simulink model "test"  (R2019b)
settings: Solver=VariableStepAuto  StartTime=0.0  StopTime=10.0  RelTol=1e-3
undefined symbols (not defined in the file or in its folder): SignalState

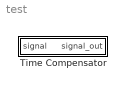
== system test ==
  Time Compensator : Subsystem  AncestorBlock=helperlibrary/Time Compensator  TreatAsAtomicUnit=on

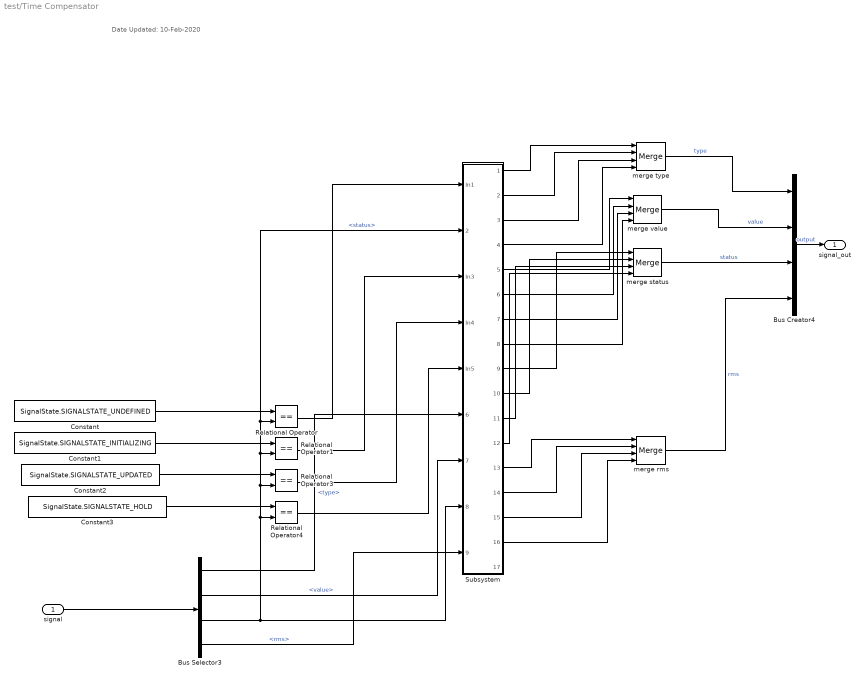
== system test/Time Compensator ==
  note: Date Updated: 10-Feb-2020
  signal : Inport
  Bus Creator4 : BusCreator  Inputs=4
  Bus Selector3 : BusSelector  OutputSignals=type,value,status,rms
  Constant : Constant  Value=SignalState.SIGNALSTATE_UNDEFINED
  Constant1 : Constant  Value=SignalState.SIGNALSTATE_INITIALIZING
  Constant2 : Constant  Value=SignalState.SIGNALSTATE_UPDATED
  Constant3 : Constant  Value=SignalState.SIGNALSTATE_HOLD
  Relational Operator{,1,3..4} (4 alike) : RelationalOperator  Operator===  OutDataTypeStr=boolean  RndMeth=Simplest
  Subsystem : Subsystem  TreatAsAtomicUnit=on
  merge rms : Merge  Inputs=4
  merge status : Merge  Inputs=4
  merge type : Merge  Inputs=4
  merge value : Merge  Inputs=4
  signal_out : Outport
  wires:
  merge type/1 -> Bus Creator4/1  "type"
  merge rms/1 -> Bus Creator4/4  "rms"
  merge value/1 -> Bus Creator4/2  "value"
  Constant3/1 -> Relational Operator4/1
  merge status/1 -> Bus Creator4/3  "status"
  Constant2/1 -> Relational Operator3/1
  Constant/1 -> Relational Operator/1
  Constant1/1 -> Relational Operator1/1
  signal/1 -> Bus Selector3/1
  Bus Creator4/1 -> signal_out/1  "output"
  Bus Selector3/3 -> Subsystem/8(<status>1), Relational Operator4/2, Relational Operator3/2, Relational Operator1/2, Subsystem/2(<status>), Relational Operator/2  "<status>"
  Relational Operator/1 -> Subsystem/1(In1)
  Relational Operator1/1 -> Subsystem/3(In3)
  Relational Operator3/1 -> Subsystem/4(In4)
  Relational Operator4/1 -> Subsystem/5(In5)
  Bus Selector3/1 -> Subsystem/6(<type>)  "<type>"
  Bus Selector3/2 -> Subsystem/7(<value>)  "<value>"
  Bus Selector3/4 -> Subsystem/9(<rms>)  "<rms>"
  Subsystem/1(Out1) -> merge type/1
  Subsystem/2(Out2) -> merge type/2
  Subsystem/3(Out3) -> merge type/3
  Subsystem/4(Out4) -> merge type/4
  Subsystem/5(Out5) -> merge value/1
  Subsystem/6(Out6) -> merge value/2
  Subsystem/7(Out7) -> merge value/3
  Subsystem/8(Out8) -> merge value/4
  Subsystem/9(Out9) -> merge status/1
  Subsystem/10(Out10) -> merge status/2
  Subsystem/11(Out11) -> merge status/3
  Subsystem/12(Out12) -> merge status/4
  Subsystem/13(Out13) -> merge rms/1
  Subsystem/14(Out14) -> merge rms/2
  Subsystem/15(Out15) -> merge rms/3
  Subsystem/16(Out16) -> merge rms/4

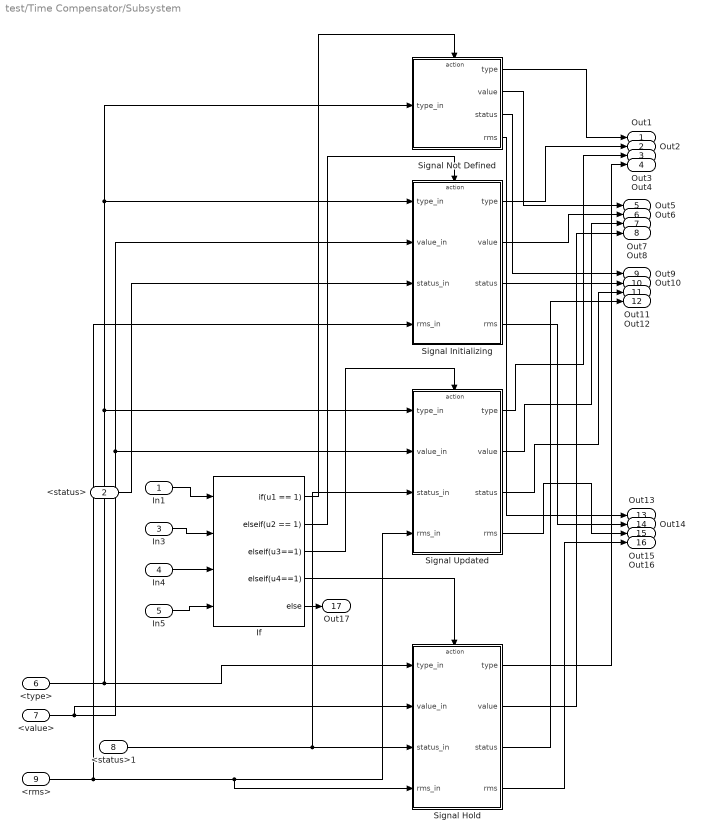
== system test/Time Compensator/Subsystem ==
  In1 : Inport
  <status> : Inport  Port=2
  In3 : Inport  Port=3
  In4 : Inport  Port=4
  In5 : Inport  Port=5
  <type> : Inport  Port=6
  <value> : Inport  Port=7
  <status>1 : Inport  Port=8
  <rms> : Inport  Port=9
  If : If  NumInputs=4  IfExpression=u1 == 1  ElseIfExpressions=u2 == 1,u3==1,u4==1
  Signal Hold : Subsystem  TreatAsAtomicUnit=on
  Signal Initializing : Subsystem  TreatAsAtomicUnit=on
  Signal Not Defined : Subsystem  TreatAsAtomicUnit=on
  Signal Updated : Subsystem  TreatAsAtomicUnit=on
  Out1 : Outport
  Out2 : Outport  Port=2
  Out3 : Outport  Port=3
  Out4 : Outport  Port=4
  Out5 : Outport  Port=5
  Out6 : Outport  Port=6
  Out7 : Outport  Port=7
  Out8 : Outport  Port=8
  Out9 : Outport  Port=9
  Out10 : Outport  Port=10
  Out11 : Outport  Port=11
  Out12 : Outport  Port=12
  Out13 : Outport  Port=13
  Out14 : Outport  Port=14
  Out15 : Outport  Port=15
  Out16 : Outport  Port=16
  Out17 : Outport  Port=17
  wires:
  <status>/1 -> Signal Initializing/3(status_in)
  Signal Initializing/3(status) -> Out10/1
  In5/1 -> If/4
  In3/1 -> If/2
  Signal Initializing/4(rms) -> Out14/1
  Signal Not Defined/2(value) -> Out5/1
  <status>1/1 -> Signal Updated/3(status_in), Signal Hold/3(status_in)
  Signal Updated/2(value) -> Out7/1
  Signal Hold/1(type) -> Out4/1
  Signal Updated/1(type) -> Out3/1
  Signal Initializing/1(type) -> Out2/1
  Signal Hold/3(status) -> Out12/1
  Signal Updated/4(rms) -> Out15/1
  Signal Not Defined/3(status) -> Out9/1
  <rms>/1 -> Signal Initializing/4(rms_in), Signal Updated/4(rms_in), Signal Hold/4(rms_in)
  Signal Hold/2(value) -> Out8/1
  In4/1 -> If/3
  Signal Initializing/2(value) -> Out6/1
  If/5 -> Out17/1
  In1/1 -> If/1
  <value>/1 -> Signal Hold/2(value_in), Signal Initializing/2(value_in), Signal Updated/2(value_in)
  Signal Not Defined/4(rms) -> Out13/1
  If/4 -> Signal Hold/Action
  If/2 -> Signal Initializing/Action
  If/1 -> Signal Not Defined/Action
  If/3 -> Signal Updated/Action
  Signal Not Defined/1(type) -> Out1/1
  Signal Updated/3(status) -> Out11/1
  Signal Hold/4(rms) -> Out16/1
  <type>/1 -> Signal Hold/1(type_in), Signal Updated/1(type_in), Signal Not Defined/1(type_in), Signal Initializing/1(type_in)

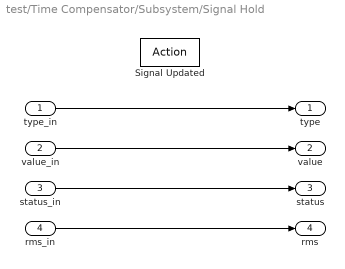
== system test/Time Compensator/Subsystem/Signal Hold ==
  type_in : Inport
  value_in : Inport  Port=2
  status_in : Inport  Port=3
  rms_in : Inport  Port=4
  Signal Updated : ActionPort  ActionPortLabel=elseif(u4==1)
  type : Outport
  value : Outport  Port=2
  status : Outport  Port=3
  rms : Outport  Port=4
  wires:
  type_in/1 -> type/1
  value_in/1 -> value/1
  rms_in/1 -> rms/1
  status_in/1 -> status/1

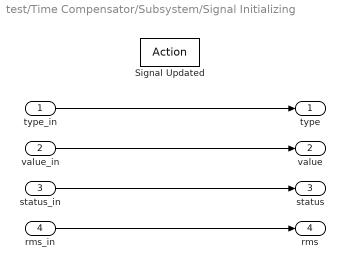
== system test/Time Compensator/Subsystem/Signal Initializing ==
  type_in : Inport
  value_in : Inport  Port=2
  status_in : Inport  Port=3
  rms_in : Inport  Port=4
  Signal Updated : ActionPort  ActionPortLabel=elseif(u2 == 1)
  type : Outport
  value : Outport  Port=2
  status : Outport  Port=3
  rms : Outport  Port=4
  wires:
  status_in/1 -> status/1
  rms_in/1 -> rms/1
  value_in/1 -> value/1
  type_in/1 -> type/1

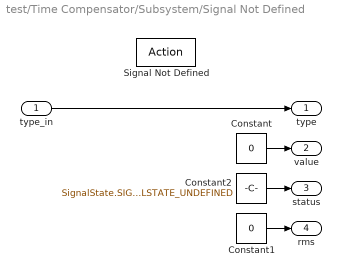
== system test/Time Compensator/Subsystem/Signal Not Defined ==
  type_in : Inport
  Signal Not Defined : ActionPort  ActionPortLabel=if(u1 == 1)
  Constant : Constant  Value=0
  Constant1 : Constant  Value=0
  Constant2 : Constant  Value=SignalState.SIGNALSTATE_UNDEFINED
  type : Outport
  value : Outport  Port=2
  status : Outport  Port=3
  rms : Outport  Port=4
  wires:
  Constant2/1 -> status/1
  Constant1/1 -> rms/1
  Constant/1 -> value/1
  type_in/1 -> type/1

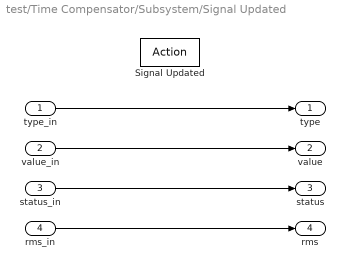
== system test/Time Compensator/Subsystem/Signal Updated ==
  type_in : Inport
  value_in : Inport  Port=2
  status_in : Inport  Port=3
  rms_in : Inport  Port=4
  Signal Updated : ActionPort  ActionPortLabel=elseif(u3==1)
  type : Outport
  value : Outport  Port=2
  status : Outport  Port=3
  rms : Outport  Port=4
  wires:
  status_in/1 -> status/1
  rms_in/1 -> rms/1
  value_in/1 -> value/1
  type_in/1 -> type/1
